simulink library "bdyFrameBuoyFnM_ul"  (R2018b)
settings: Solver=VariableStepAuto  StartTime=0.0  StopTime=10.0  RelTol=1e-3
undefined symbols (not defined in the file): grav, Rcb_cm, rho_fluid, vol
libraries: vrlib x1, eulAng2RotMat_ul x1
settings Model: Creator=Ayaz  LastModifiedBy=Ayaz

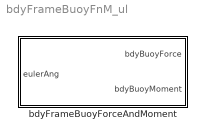
== system bdyFrameBuoyFnM_ul ==
  bdyFrameBuoyForceAndMoment : Subsystem  mask{vol=vol, rho_fluid=rho_fluid, g=grav, Rcb_cm=Rcb_cm}
      mask prompts: vol "Body volume"; rho_fluid "Fluid density"; g "Gravitation acceleration"; Rcb_cm "Center of buoyamcy vector"

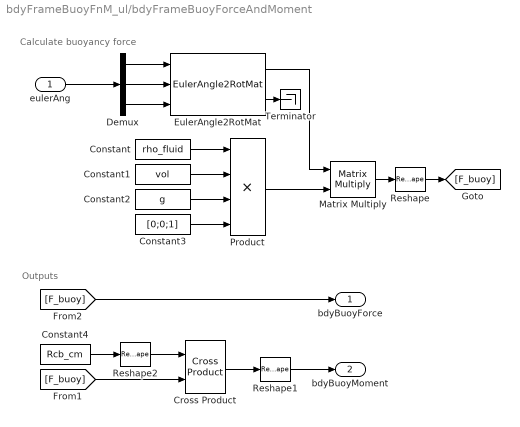
== system bdyFrameBuoyFnM_ul/bdyFrameBuoyForceAndMoment ==
  note: Calculate buoyancy force
  note: Outputs
  eulerAng : Inport
  Constant : Constant  Value=rho_fluid
  Constant1 : Constant  Value=vol
  Constant2 : Constant  Value=g
  Constant3 : Constant  Value=[0;0;1]  VectorParams1D=off
  Constant4 : Constant  Value=Rcb_cm  VectorParams1D=off
  Cross Product : vrlib/Utilities/Cross Product
      settings: SourceProductBaseCode=VR
  Demux : Demux  Outputs=3
  EulerAngle2RotMat : eulAng2RotMat_ul/EulerAngle2RotMat  SystemSampleTime=-1
  Matrix Multiply : Product  Multiplication=Matrix(*)
  Product : Product  Inputs=4
  Reshape : Reshape  OutputDimensionality=Column vector (2-D)
  Reshape1 : Reshape  OutputDimensionality=Column vector (2-D)
  Reshape2 : Reshape  OutputDimensionality=Column vector (2-D)
  Terminator : Terminator
  bdyBuoyForce : Outport
  bdyBuoyMoment : Outport  Port=2
  wires:
  eulerAng/1 -> Demux/1
  Demux/1 -> EulerAngle2RotMat/1
  Demux/2 -> EulerAngle2RotMat/2
  Demux/3 -> EulerAngle2RotMat/3
  Constant3/1 -> Product/4
  Constant2/1 -> Product/3
  Constant1/1 -> Product/2
  Constant/1 -> Product/1
  EulerAngle2RotMat/2 -> Terminator/1
  EulerAngle2RotMat/1 -> Matrix Multiply/1
  Product/1 -> Matrix Multiply/2
  Matrix Multiply/1 -> Reshape/1
  Reshape/1 -> [F_buoy]
  [F_buoy] -> bdyBuoyForce/1
  [F_buoy] -> Cross Product/2
  Reshape1/1 -> bdyBuoyMoment/1
  Cross Product/1 -> Reshape1/1
  Constant4/1 -> Reshape2/1
  Reshape2/1 -> Cross Product/1
